simulink model "MPC_sim"  (R2018b)
settings: Solver=VariableStepAuto  StartTime=0.0  StopTime=200  RelTol=1e-3
values from neighbouring files (symbols this model uses):
  A = [0 1;0 0]    [MPC.m]    (also in alt_identif.m)
  Ad = (eye(length(sys_s.A)) + sys_s.A*Ts)    [MPC.m]    (also in alt_identif.m)
  Ad_aug = [Ad Bd; zeros(1,length(Ad)) 1]    [MPC.m]
  B = [0;1/m]    [MPC.m]    (also in alt_identif.m)
  Bd = sys_s.B*Ts    [MPC.m]    (also in alt_identif.m)
  Bd_aug = [Bd;1]    [MPC.m]
  Bm = Bm * 4    [MPC.m]    (also in alt_identif.m = Bm)
  C = [1 0]    [MPC.m]    (also in alt_identif.m)
  Cd = sys_s.C    [MPC.m]    (also in alt_identif.m)
  Cd_aug = [Cd 0]    [MPC.m]
  D = [0]    [MPC.m]    (also in alt_identif.m)
  g = 9.8    [MPC.m]    (also in alt_identif.m)
  sys_s = series(sys1,sys2)    [MPC.m]    (also in alt_identif.m)
  Ts = 1/5    (= 0.2)    [MPC.m]    (also in alt_identif.m; motor_model_fin.m)
undefined symbols (not defined in the file or in its folder): Am, Cm, DiscIntNeverNeededParam, Dm
libraries: simulink x2
settings Model: Creator=Dragos  LastModifiedBy=Dragos
settings SolverCC: AlgebraicLoopSolver=LineSearch

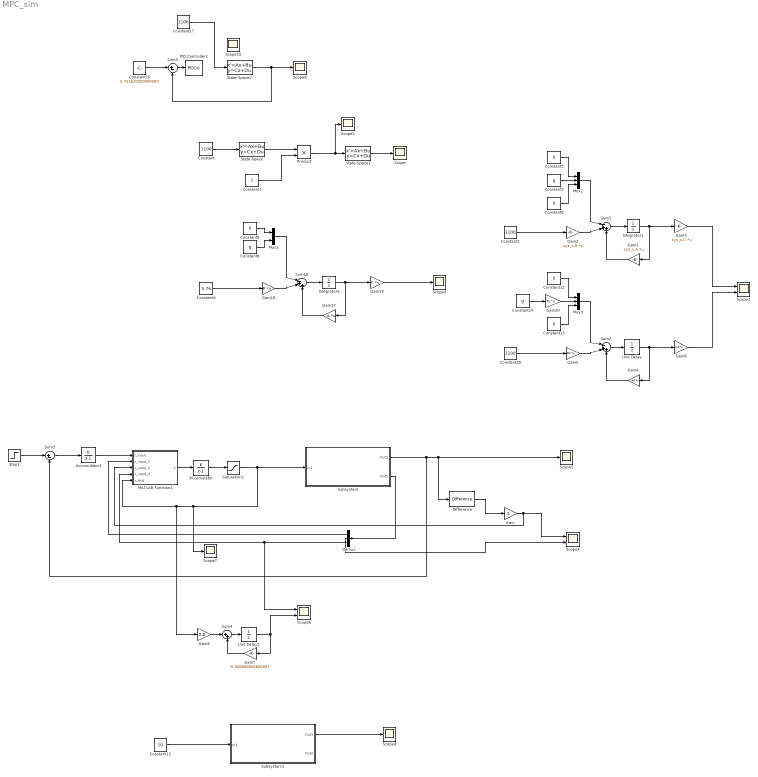
== system MPC_sim ==
  Accumulator : DiscreteIntegrator  IntegratorMethod=Accumulation: Forward Euler  SampleTime=-1  ICPrevOutput=DiscIntNeverNeededParam  ICPrevScaledInput=DiscIntNeverNeededParam
  Accumulator2 : DiscreteIntegrator  IntegratorMethod=Accumulation: Forward Euler  gainval=0.01  SampleTime=-1  ICPrevOutput=DiscIntNeverNeededParam  ICPrevScaledInput=DiscIntNeverNeededParam
  Constant : Constant  Value=1100
  Constant1 : Constant
  Constant10 : Constant  Value=1100
  Constant{5..6,9,12..13} (5 alike) : Constant  Value=0
  Constant14 : Constant  Value=g
  Constant15 : Constant  Value=10
  Constant16 : Constant  Value=5.751620000000000
  Constant17 : Constant  Value=1106
  Constant2 : Constant  Value=1100
  Constant3 : Constant  Value=g
  Constant4 : Constant  Value=5.76
  Constant8 : Constant  Value=g
  Demux : Demux  Outputs=3
  Difference : simulink/Discrete/Difference  ICPrevInput=0.0  OutMin=[]  OutMax=[]  OutDataType=fixdt(1, 16)  OutScaling=2^-10  DoSatur=off
  Gain : Gain  Gain=5
  Gain1 : Gain  Gain=sys_s.A  Multiplication=Matrix(K*u)
  Gain17 : Gain  Gain=A  Multiplication=Matrix(K*u)
  Gain18 : Gain  Gain=B  Multiplication=Matrix(K*u)
  Gain19 : Gain  Gain=C  Multiplication=Matrix(K*u)
  Gain2 : Gain  Gain=sys_s.B  Multiplication=Matrix(K*u)
  Gain20 : Gain  Gain=Ts  Multiplication=Matrix(K*u)
  Gain3 : Gain  Gain=sys_s.C  Multiplication=Matrix(K*u)
  Gain4 : Gain  Gain=Ad  Multiplication=Matrix(K*u)
  Gain5 : Gain  Gain=Bd  Multiplication=Matrix(K*u)
  Gain6 : Gain  Gain=Cd  Multiplication=Matrix(K*u)
  Gain7 : Gain  Gain=-0.666666666666667
  Gain8 : Gain  Gain=0.8
  Integrator1 : Integrator  InitialCondition=[0 0 0]
  Integrator5 : Integrator  InitialCondition=[0 0]
  MATLAB Function1 : MATLAB Function  TreatAsAtomicUnit=on
  Mux1 : Mux  Inputs=3
  Mux2 : Mux  Inputs=2
  Mux3 : Mux  Inputs=3
  PID Controller1 : simulink/Continuous/PID Controller  Controller=PID  Form=Parallel  TimeDomain=Continuous-time  SampleTime=-1  IntegratorMethod=Forward Euler  FilterMethod=Forward Euler  ControllerParametersSource=internal  P=257.226983422135  I=4284.53920903726  D=-1.12098211406954  UseFilter=on  N=31.5078470985719  TunerSelectOption=Transfer Function Based (PID Tuner App)  InitialConditionSource=internal  InitialConditionForIntegrator=0  InitialConditionForFilter=0  DifferentiatorICPrevScaledInput=0  ExternalReset=none  TrackingMode=off  Kt=1  LimitOutput=off  UpperSaturationLimit=inf  LowerSaturationLimit=-inf  LinearizeAsGain=on  AntiWindupMode=none  Kb=1  POutMin=[]  POutMax=[]  IOutMin=[]  IOutMax=[]  DOutMin=[]  DOutMax=[]  NOutMin=[]  NOutMax=[]  SumOutMin=[]  SumOutMax=[]  SaturationOutMin=[]  SaturationOutMax=[]  PParamMin=[]  PParamMax=[]  IParamMin=[]  IParamMax=[]  DParamMin=[]  DParamMax=[]  NParamMin=[]  NParamMax=[]  KbParamMin=[]  KbParamMax=[]  KtParamMin=[]  KtParamMax=[]  KbOutMin=[]  KbOutMax=[]  KtOutMin=[]  KtOutMax=[]  IntegratorOutMin=[]  IntegratorOutMax=[]  FilterOutMin=[]  FilterOutMax=[]  SumI1OutMin=[]  SumI1OutMax=[]  SumI2OutMin=[]  SumI2OutMax=[]  SumI3OutMin=[]  SumI3OutMax=[]  SumI4OutMin=[]  SumI4OutMax=[]  SumDOutMin=[]  SumDOutMax=[]  DifferentiatorOutMin=[]  DifferentiatorOutMax=[]  FilterDiffOutCoefMin=[]  FilterDiffOutCoefMax=[]  ReciprocalOutMin=[]  ReciprocalOutMax=[]  SumDenOutMin=[]  SumDenOutMax=[]  SumNumOutMin=[]  SumNumOutMax=[]  DivideOutMin=[]  DivideOutMax=[]  IntegratorContinuousStateAttributes=''  IntegratorStateMustResolveToSignalObject=off  IntegratorRTWStateStorageClass=Auto  FilterContinuousStateAttributes=''  FilterStateMustResolveToSignalObject=off  FilterRTWStateStorageClass=Auto  ParallelPVariant=InternalParameters  IdealPVariant=Disabled  IVariant=InternalParameters  DVariant=InternalParameters  IntegratorVariant=Continuous  SatVariant=Disabled  AWVariant=Passthrough  PCopyVariant=Disabled  TRVariant=Disabled  FdbkBlocksVariant=Forward  IdealPFdbkVariant=Disabled  SatFdbkVariant=Disabled  DerivativeFilterVariant=ContFilter  NVariant=InternalParameters  NCopyVariant=Disabled  FilterICVariant=InternalICsFilter  IntegratorICVariant=InternalICs  ExternalResetVariant=Disabled  TRSumVariant=Passthrough  SumFdbkVariant=Disabled  SumVariant=Sum_PID
  Product : Product
  Saturation1 : Saturate  UpperLimit=3000  LowerLimit=0
  Scope{,1,3,5,7..10} (8 alike) : Scope
  Scope2 : Scope  NumInputPorts=2
  Scope4 : Scope  NumInputPorts=2
  Scope6 : Scope  NumInputPorts=2
  State-Space : StateSpace  A=Am  B=Bm  C=Cm  D=Dm  InitialCondition=0
  State-Space1 : StateSpace  A=A  B=B  C=C  D=D  InitialCondition=0
  State-Space2 : StateSpace  A=Am  B=Bm  C=Cm  D=Dm  InitialCondition=0
  Step1 : Step  Time=500  Before=0.1  After=20  SampleTime=0
  Subsystem : Subsystem
  Subsystem1 : Subsystem
  Sum1 : Sum  Inputs=|-++
  Sum10 : Sum  Inputs=|-++
  Sum2 : Sum  Inputs=|-++
  Sum3 : Sum  Inputs=|+-
  Sum4 : Sum  Inputs=|++
  Sum5 : Sum  Inputs=|+-
  Unit Delay : UnitDelay  InitialCondition=[0 0 0]  SampleTime=Ts
  Unit Delay1 : UnitDelay  InitialCondition=[0]  SampleTime=Ts
  wires:
  Constant/1 -> State-Space/1
  State-Space/1 -> Product/1
  Constant1/1 -> Product/2
  Product/1 -> Scope1/1, State-Space1/1
  State-Space1/1 -> Scope/1
  Constant9/1 -> Mux2/1
  Integrator5/1 -> Gain17/1, Gain19/1
  Constant8/1 -> Mux2/2
  Gain19/1 -> Scope3/1
  Gain17/1 -> Sum10/3
  Gain18/1 -> Sum10/2
  Sum10/1 -> Integrator5/1
  Constant4/1 -> Gain18/1
  Sum1/1 -> Integrator1/1
  Gain1/1 -> Sum1/3
  Gain3/1 -> Scope2/1
  Gain2/1 -> Sum1/2
  Constant3/1 -> Mux1/2
  Constant2/1 -> Gain2/1
  Mux1/1 -> Sum1/1
  Integrator1/1 -> Gain1/1, Gain3/1
  Constant5/1 -> Mux1/1
  Constant6/1 -> Mux1/3
  Mux2/1 -> Sum10/1
  Mux3/1 -> Sum2/1
  Constant10/1 -> Gain5/1
  Gain4/1 -> Sum2/3
  Gain6/1 -> Scope2/2
  Unit Delay/1 -> Gain4/1, Gain6/1
  Gain5/1 -> Sum2/2
  Constant13/1 -> Mux3/3
  Sum2/1 -> Unit Delay/1
  Gain20/1 -> Mux3/2
  Constant12/1 -> Mux3/1
  Constant14/1 -> Gain20/1
  Subsystem/1(Out1) -> Scope5/1, Difference/1, Sum5/2
  Constant15/1 -> Subsystem1/1(In1)
  Subsystem1/1(Out1) -> Scope8/1
  MATLAB Function1/1(y) -> Accumulator/1
  Constant16/1 -> Sum3/1
  State-Space2/1 -> Sum3/2, Scope9/1
  Sum3/1 -> PID Controller1/1
  Constant17/1 -> State-Space2/1
  Accumulator/1 -> Saturation1/1
  Step1/1 -> Sum5/1
  Sum5/1 -> Accumulator2/1
  Accumulator2/1 -> MATLAB Function1/1(r_input)
  Saturation1/1 -> Subsystem/1(In1), Scope7/1, Gain8/1, MATLAB Function1/5(x_aug)
  Subsystem/2(Out2) -> Demux/1
  Demux/2 -> Scope4/2
  Demux/3 -> Scope6/1, MATLAB Function1/4(x_input_3)
  Difference/1 -> Gain/1
  Gain/1 -> MATLAB Function1/3(x_input_2), Scope4/1
  Unit Delay1/1 -> Gain7/1, Scope6/2
  Gain8/1 -> Sum4/1
  Sum4/1 -> Unit Delay1/1
  Gain7/1 -> Sum4/2
  Demux/1 -> MATLAB Function1/2(x_input_1)

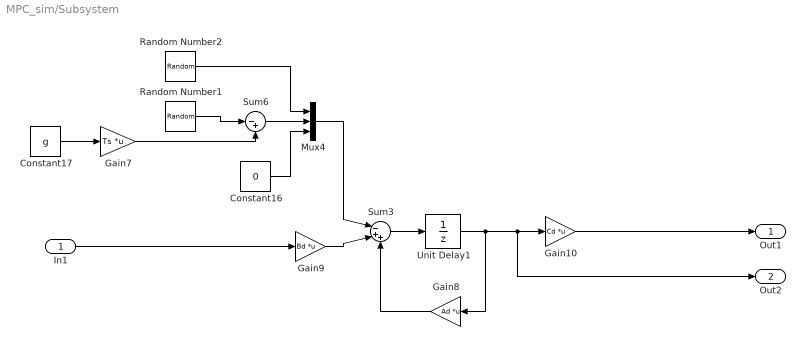
== system MPC_sim/Subsystem ==
  In1 : Inport
  Constant16 : Constant  Value=0
  Constant17 : Constant  Value=g
  Gain10 : Gain  Gain=Cd  Multiplication=Matrix(K*u)
  Gain7 : Gain  Gain=Ts  Multiplication=Matrix(K*u)
  Gain8 : Gain  Gain=Ad  Multiplication=Matrix(K*u)
  Gain9 : Gain  Gain=Bd  Multiplication=Matrix(K*u)
  Mux4 : Mux  Inputs=3
  Random Number1 : RandomNumber  Variance=0.01  Seed=142753  SampleTime=Ts
  Random Number2 : RandomNumber  Variance=0  Seed=142753  SampleTime=Ts
  Sum3 : Sum  Inputs=|-++
  Sum6 : Sum  Inputs=|-+
  Unit Delay1 : UnitDelay  InitialCondition=[0 0 0]  SampleTime=Ts
  Out1 : Outport
  Out2 : Outport  Port=2
  wires:
  Random Number2/1 -> Mux4/1
  Sum3/1 -> Unit Delay1/1
  Mux4/1 -> Sum3/1
  Constant16/1 -> Mux4/3
  Unit Delay1/1 -> Gain8/1, Gain10/1, Out2/1
  Constant17/1 -> Gain7/1
  Gain8/1 -> Sum3/3
  Gain9/1 -> Sum3/2
  In1/1 -> Gain9/1
  Gain10/1 -> Out1/1
  Sum6/1 -> Mux4/2
  Gain7/1 -> Sum6/2
  Random Number1/1 -> Sum6/1

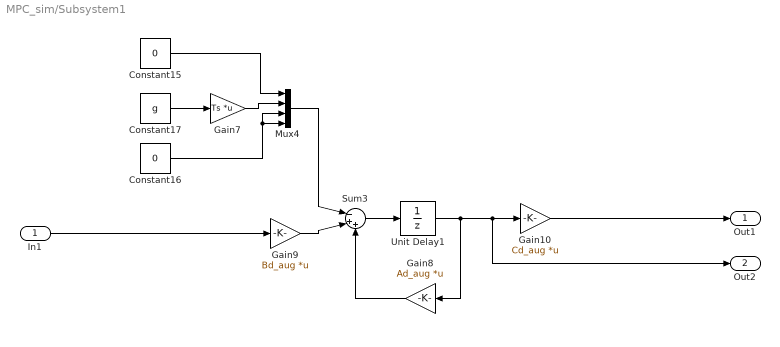
== system MPC_sim/Subsystem1 ==
  In1 : Inport
  Constant15 : Constant  Value=0
  Constant16 : Constant  Value=0
  Constant17 : Constant  Value=g
  Gain10 : Gain  Gain=Cd_aug  Multiplication=Matrix(K*u)
  Gain7 : Gain  Gain=Ts  Multiplication=Matrix(K*u)
  Gain8 : Gain  Gain=Ad_aug  Multiplication=Matrix(K*u)
  Gain9 : Gain  Gain=Bd_aug  Multiplication=Matrix(K*u)
  Mux4 : Mux
  Sum3 : Sum  Inputs=|-++
  Unit Delay1 : UnitDelay  InitialCondition=[0 0 0 0]  SampleTime=Ts
  Out1 : Outport
  Out2 : Outport  Port=2
  wires:
  Gain7/1 -> Mux4/2
  Constant15/1 -> Mux4/1
  Sum3/1 -> Unit Delay1/1
  Mux4/1 -> Sum3/1
  Constant16/1 -> Mux4/4, Mux4/3
  Unit Delay1/1 -> Gain8/1, Gain10/1, Out2/1
  Constant17/1 -> Gain7/1
  Gain8/1 -> Sum3/3
  Gain9/1 -> Sum3/2
  In1/1 -> Gain9/1
  Gain10/1 -> Out1/1

== matlab function MPC_sim/MATLAB Function1 ==
  data: r_input input; x_input_1 input; x_input_2 input; x_input_3 input; y output; x_aug input
function y= fcn(r_input,x_input_1,x_input_2,x_input_3,x_aug)
    Ad = [1 0.2 0;0 1 0.00177777777777778;0 0 -0.666666666666667];
    Bd = [0;0;0.2];
    Cd = [1 0 0];

    Ad_aug = [Ad Bd; zeros(1,length(Ad)) 1];
    Bd_aug = [Bd;1];
    Cd_aug = [Cd 0];


    Q=100;
    R=1;
    S=100;
    hz=100;

    CQC = Cd_aug'*Q*Cd_aug;
    CSC = Cd_aug'*Q*Cd_aug;
    QC = Q*Cd_aug;
    SC = S*Cd_aug;

    Qdb = zeros(length(CQC)*hz,length(CQC)*hz);
    Rdb = zeros(hz,hz);
    Tdb = zeros(hz,length(CQC)*hz);
    Cdb = zeros(length(Bd_aug)*hz,hz);
    Adc = zeros(hz*length(Ad_aug),length(Ad_aug));

    for i=1:hz
        i_begin = (i-1)*length(CQC)+1;
        i_end = i*length(CQC);

        if i<hz
            Qdb(i_begin:i_end,i_begin:i_end) = CQC;
            Tdb(i,i_begin:i_end) = QC;
        else
            Qdb(i_begin:i_end,i_begin:i_end) = CSC;
            Tdb(i,i_begin:i_end) = SC;
        end

        Rdb(i,i) = R;
        Adc((i-1)*length(Ad_aug)+1:i*length(Ad_aug),1:length(Ad_aug)) = Ad_aug^i;

        for j=1:hz
            if j<=i
                Cdb((i-1)*length(Bd_aug)+1:i*length(Bd_aug),j) = Ad_aug^(i-j)*Bd_aug;
            end
        end
    end%4.8614

    Hdb = Cdb'*Qdb*Cdb + Rdb;
    Fdbt = [Adc'*Qdb*Cdb;-Tdb*Cdb];

    x = [x_input_1;x_input_2;x_input_3; x_aug];
    r = ones(1,100)*r_input;

    ft = [x' r]*Fdbt
    du=-inv(Hdb)*ft'
    
    y = du(1)
end
